simulink model "harmonic"  (R2021b)
settings: Solver=VariableStepAuto  StartTime=0.0  StopTime=15.0  RelTol=1e-3
settings Model: Creator=iliya122  LastModifiedBy=Ivan
settings SolverCC: AlgebraicLoopSolver=TrustRegion
settings DebuggingCC: SFMachineParentedDataDiag=warning

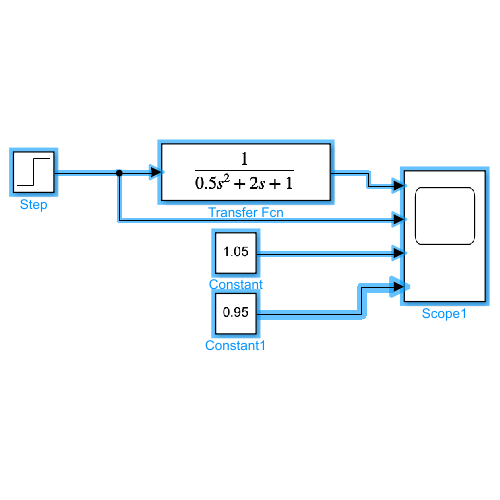
[thumbnail: Simulink's stored preview of the top-level diagram]
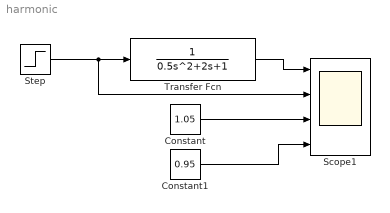
== system harmonic ==
  Constant : Constant  Value=1.05
  Constant1 : Constant  Value=0.95
  Scope1 : Scope  NumInputPorts=4
  Step : Step  Time=2  SampleTime=0
  Transfer Fcn : TransferFcn  Numerator=1  Denominator=[0.5 2 1]
  wires:
  Constant/1 -> Scope1/3
  Step/1 -> Transfer Fcn/1, Scope1/2
  Constant1/1 -> Scope1/4
  Transfer Fcn/1 -> Scope1/1
